simulink model "IM_Open_Loop"  (R2019b)
settings: Solver=VariableStepAuto  StartTime=0.0  StopTime=2  RelTol=1e-3
values from neighbouring files (symbols this model uses):
  B = 0.068    [IM_Model_Parameters.m]
  fn = 50    [IM_Model_Parameters.m]
  J = 0.4    [IM_Model_Parameters.m]
  Lks = Ls - Lm^2/Lr    (= 0.00442538071066)    [IM_Model_Parameters.m]
  Lm = 57e-3    (= 0.057)    [IM_Model_Parameters.m]
  np = 3    [IM_Model_Parameters.m]
  Rr = 0.175    [IM_Model_Parameters.m]
  Rs = 0.24    [IM_Model_Parameters.m]
  vsat = 380    [IM_Model_Parameters.m]
settings Model: Creator=hassancurrimbhoy  LastModifiedBy=hassancurrimbhoy
settings SolverCC: ZeroCrossAlgorithm=Adaptive

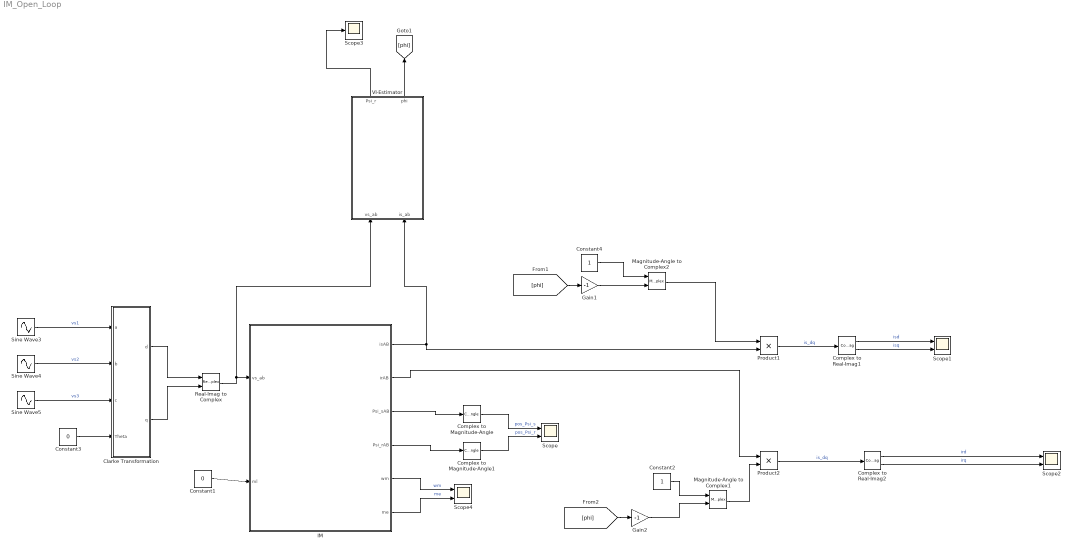
== system IM_Open_Loop ==
  Clarke Transformation : Subsystem
  Complex to Magnitude-Angle : ComplexToMagnitudeAngle  Output=Angle
  Complex to Magnitude-Angle1 : ComplexToMagnitudeAngle  Output=Angle
  Complex to Real-Imag1 : ComplexToRealImag
  Complex to Real-Imag2 : ComplexToRealImag
  Constant1 : Constant  Value=0
  Constant2 : Constant
  Constant3 : Constant  Value=0
  Constant4 : Constant
  Gain1 : Gain  Gain=-1
  Gain2 : Gain  Gain=-1
  IM : Subsystem
      mask Display: image('$imagefile'); % Use "Edit Image" on toolstrip to change.
  Magnitude-Angle to Complex1 : MagnitudeAngleToComplex
  Magnitude-Angle to Complex2 : MagnitudeAngleToComplex
  Product1 : Product
  Product2 : Product
  Real-Imag to Complex : RealImagToComplex
  Scope{,1..2,4} (4 alike) : Scope  NumInputPorts=2
  Scope3 : Scope
  Sine Wave3 : Sin  Amplitude=vsat  Frequency=2*pi*fn  SampleTime=0
  Sine Wave4 : Sin  Amplitude=vsat  Frequency=2*pi*fn  Phase=-2*pi/3  SampleTime=0
  Sine Wave5 : Sin  Amplitude=vsat  Frequency=2*pi*fn  Phase=-4*pi/3  SampleTime=0
  VI-Estimator : Subsystem
  wires:
  Sine Wave5/1 -> Clarke Transformation/3(c)  "vs3"
  Sine Wave4/1 -> Clarke Transformation/2("b ")  "vs2"
  Clarke Transformation/1(d) -> Real-Imag to Complex/1
  Clarke Transformation/2(q) -> Real-Imag to Complex/2
  Real-Imag to Complex/1 -> VI-Estimator/1(vs_ab), IM/1(vs_ab)
  Constant3/1 -> Clarke Transformation/4(Theta)
  IM/5(wm) -> Scope4/1  "wm"
  IM/6(me) -> Scope4/2  "me"
  Constant1/1 -> IM/2(ml)
  Constant4/1 -> Magnitude-Angle to Complex2/1
  Gain1/1 -> Magnitude-Angle to Complex2/2
  [phi] -> Gain1/1
  Product1/1 -> Complex to Real-Imag1/1  "is_dq"
  Magnitude-Angle to Complex2/1 -> Product1/1
  Complex to Real-Imag1/1 -> Scope1/1  "isd"
  Complex to Real-Imag1/2 -> Scope1/2  "isq"
  IM/1(isAB) -> Product1/2, VI-Estimator/2(is_ab)
  VI-Estimator/2(phi) -> [phi]
  VI-Estimator/1(Psi_r) -> Scope3/1
  Gain2/1 -> Magnitude-Angle to Complex1/2
  Product2/1 -> Complex to Real-Imag2/1  "is_dq"
  Complex to Real-Imag2/1 -> Scope2/1  "ird"
  Complex to Real-Imag2/2 -> Scope2/2  "irq"
  Magnitude-Angle to Complex1/1 -> Product2/2
  IM/2(irAB) -> Product2/1
  [phi] -> Gain2/1
  Constant2/1 -> Magnitude-Angle to Complex1/1
  Sine Wave3/1 -> Clarke Transformation/1(a)  "vs1"
  Complex to Magnitude-Angle/1 -> Scope/1  "pos_Psi_s"
  IM/3(Psi_sAB) -> Complex to Magnitude-Angle/1
  IM/4(Psi_rAB) -> Complex to Magnitude-Angle1/1
  Complex to Magnitude-Angle1/1 -> Scope/2  "pos_Psi_r"

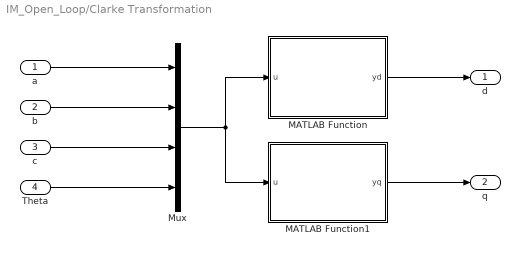
== system IM_Open_Loop/Clarke Transformation ==
  a : Inport
  "b " : Inport  Port=2
  c : Inport  Port=3
  Theta : Inport  Port=4
  MATLAB Function : MATLAB Function  TreatAsAtomicUnit=on
  MATLAB Function1 : MATLAB Function  TreatAsAtomicUnit=on
  Mux : Mux
  d : Outport
  q : Outport  Port=2
  wires:
  "b "/1 -> Mux/2
  Theta/1 -> Mux/4
  MATLAB Function1/1(yq) -> q/1
  MATLAB Function/1(yd) -> d/1
  c/1 -> Mux/3
  Mux/1 -> MATLAB Function1/1(u), MATLAB Function/1(u)
  a/1 -> Mux/1

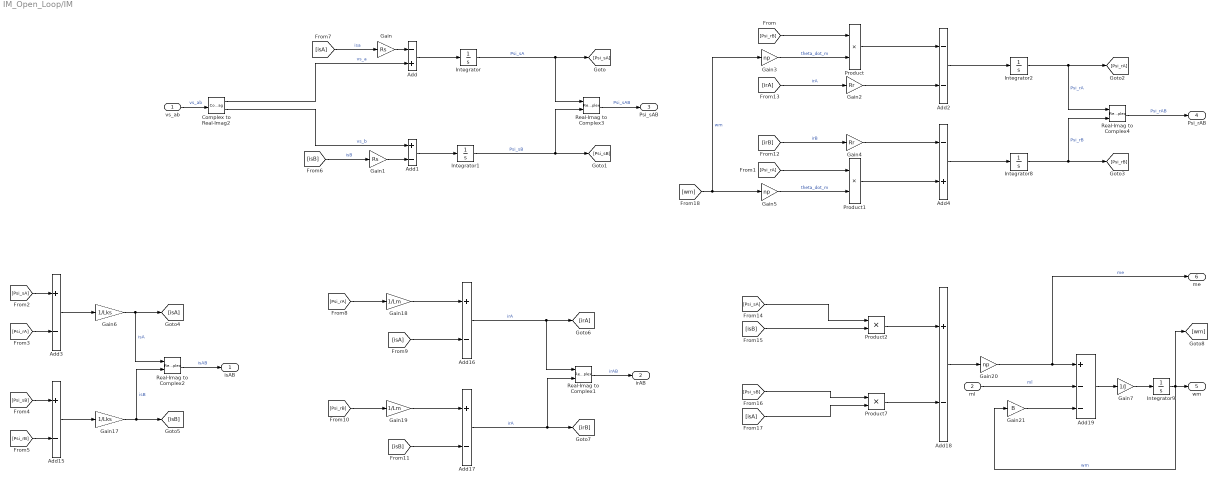
== system IM_Open_Loop/IM ==
  vs_ab : Inport
  ml : Inport  Port=2
  Add : Sum  Inputs=-+
  Add{1,3,15..18} (6 alike) : Sum  Inputs=+-
  Add19 : Sum  Inputs=+--
  Add2 : Sum  Inputs=--
  Add4 : Sum  Inputs=-+
  Complex to Real-Imag2 : ComplexToRealImag
  Gain : Gain  Gain=Rs
  Gain1 : Gain  Gain=Rs
  Gain17 : Gain  Gain=1/Lks
  Gain18 : Gain  Gain=1/Lm
  Gain19 : Gain  Gain=1/Lm
  Gain2 : Gain  Gain=Rr
  Gain20 : Gain  Gain=np
  Gain21 : Gain  Gain=B
  Gain3 : Gain  Gain=np
  Gain4 : Gain  Gain=Rr
  Gain5 : Gain  Gain=np
  Gain6 : Gain  Gain=1/Lks
  Gain7 : Gain  Gain=1/J
  Integrator{,1..2,8..9} (5 alike) : Integrator
  Product{,1..2,7} (4 alike) : Product
  Real-Imag to Complex{1..4} (4 alike) : RealImagToComplex
  isAB : Outport
  irAB : Outport  Port=2
  Psi_sAB : Outport  Port=3
  Psi_rAB : Outport  Port=4
  wm : Outport  Port=5
  me : Outport  Port=6
  wires:
  vs_ab/1 -> Complex to Real-Imag2/1  "vs_ab"
  Complex to Real-Imag2/1 -> Add/2  "vs_a"
  Complex to Real-Imag2/2 -> Add1/1  "vs_b"
  [isA] -> Gain/1  "isa"
  Add/1 -> Integrator/1
  Integrator/1 -> [Psi_sA], Real-Imag to Complex3/1  "Psi_sA"
  Add1/1 -> Integrator1/1
  [isB] -> Gain1/1  "isB"
  Gain1/1 -> Add1/2
  Integrator1/1 -> Real-Imag to Complex3/2, [Psi_sB]  "Psi_sB"
  Real-Imag to Complex3/1 -> Psi_sAB/1  "Psi_sAB"
  Integrator2/1 -> Real-Imag to Complex4/1, [Psi_rA]  "Psi_rA"
  Integrator8/1 -> [Psi_rB], Real-Imag to Complex4/2  "Psi_rB"
  Real-Imag to Complex4/1 -> Psi_rAB/1  "Psi_rAB"
  Add2/1 -> Integrator2/1
  Add4/1 -> Integrator8/1
  Product/1 -> Add2/1
  Gain2/1 -> Add2/2
  [irA] -> Gain2/1  "irA"
  [Psi_rB] -> Product/1
  Gain3/1 -> Product/2  "theta_dot_m"
  Gain/1 -> Add/1
  Gain4/1 -> Add4/1
  [irB] -> Gain4/1  "irB"
  [wm] -> Gain3/1, Gain5/1  "wm"
  [Psi_rA] -> Product1/1
  Product1/1 -> Add4/2
  Gain5/1 -> Product1/2  "theta_dot_m"
  Add3/1 -> Gain6/1
  Gain6/1 -> Real-Imag to Complex2/1, [isA]  "isA"
  [Psi_sA] -> Add3/1
  [Psi_rA] -> Add3/2
  [Psi_rB] -> Add15/2
  Add15/1 -> Gain17/1
  [Psi_sB] -> Add15/1
  Gain17/1 -> Real-Imag to Complex2/2, [isB]  "isB"
  Add16/1 -> Real-Imag to Complex1/1, [irA]  "irA"
  Gain18/1 -> Add16/1
  [Psi_rA] -> Gain18/1
  [isA] -> Add16/2
  Add17/1 -> Real-Imag to Complex1/2, [irB]  "irA"
  Gain19/1 -> Add17/1
  [Psi_rB] -> Gain19/1
  [isB] -> Add17/2
  Gain20/1 -> me/1, Add19/1  "me"
  Product7/1 -> Add18/2
  Product2/1 -> Add18/1
  Gain21/1 -> Add19/3
  Add18/1 -> Gain20/1
  Integrator9/1 -> [wm], Gain21/1, wm/1  "wm"
  ml/1 -> Add19/2  "ml"
  [Psi_sA] -> Product2/1
  [isB] -> Product2/2
  [Psi_sB] -> Product7/1
  [isA] -> Product7/2
  Real-Imag to Complex1/1 -> irAB/1  "irAB"
  Real-Imag to Complex2/1 -> isAB/1  "isAB"
  Add19/1 -> Gain7/1
  Gain7/1 -> Integrator9/1

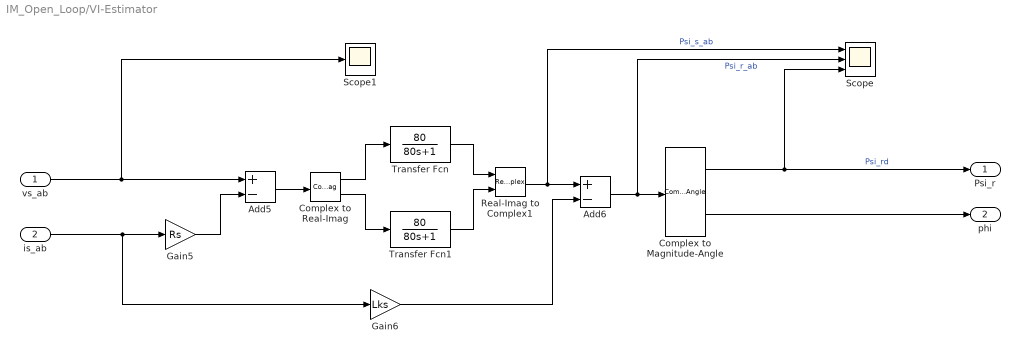
== system IM_Open_Loop/VI-Estimator ==
  vs_ab : Inport
  is_ab : Inport  Port=2
  Add5 : Sum  Inputs=+-
  Add6 : Sum  Inputs=+-
  Complex to Magnitude-Angle : ComplexToMagnitudeAngle
  Complex to Real-Imag : ComplexToRealImag
  Gain5 : Gain  Gain=Rs
  Gain6 : Gain  Gain=Lks
  Real-Imag to Complex1 : RealImagToComplex
  Scope : Scope  NumInputPorts=3
  Scope1 : Scope
  Transfer Fcn : TransferFcn  Numerator=[80]  Denominator=[80 1]
  Transfer Fcn1 : TransferFcn  Numerator=[80]  Denominator=[80 1]
  Psi_r : Outport
  phi : Outport  Port=2
  wires:
  vs_ab/1 -> Scope1/1, Add5/1
  Gain5/1 -> Add5/2
  Complex to Magnitude-Angle/1 -> Scope/3, Psi_r/1  "Psi_rd"
  Add6/1 -> Scope/2, Complex to Magnitude-Angle/1  "Psi_r_ab"
  Gain6/1 -> Add6/2
  Real-Imag to Complex1/1 -> Scope/1, Add6/1  "Psi_s_ab"
  Add5/1 -> Complex to Real-Imag/1
  is_ab/1 -> Gain6/1, Gain5/1
  Complex to Magnitude-Angle/2 -> phi/1
  Complex to Real-Imag/2 -> Transfer Fcn1/1
  Transfer Fcn1/1 -> Real-Imag to Complex1/2
  Complex to Real-Imag/1 -> Transfer Fcn/1
  Transfer Fcn/1 -> Real-Imag to Complex1/1

== matlab function IM_Open_Loop/Clarke Transformation/MATLAB Function ==
  data: u input; yd output
function yd= f(u)

yd = 2/3*(u(1)*cos(u(4)) + u(2)*cos(u(4)-2/3*pi) + u(3)*cos(u(4)-4/3*pi));

== matlab function IM_Open_Loop/Clarke Transformation/MATLAB Function1 ==
  data: u input; yq output
function yq = f(u)

yq = 2/3*(-u(1)*sin(u(4)) - u(2)*sin(u(4)-2/3*pi) - u(3)*sin(u(4)+2/3*pi));
